simulink model "TBS_SIM"  (R2016b)
settings: Solver=ode5  StartTime=15  StopTime=30  FixedStep=0.002  RelTol=1e-3
PreLoadFcn:
  | TBS_Cai_simu_init_20170316
InitFcn:
  | TBS_Cai_simu_init_20170214
StopFcn:
  | TBS_SIMULATION_LOG
undefined symbols (not defined in the file): air_density, L1X, L2X, L3X, L3Y, MAC1, MAC2, MAC3, magnitude, motor_m0, motor_t0, ORIGIN_CD, ORIGIN_CL, ORIGIN_CM, S_seg1, S_seg2, S_seg3, y_ac
libraries: aerolibconvert2 x20, simulink x13, aerolibtransform2 x4, aerolibwind2 x3, aerolib6dof2 x1, aerolibasang x1
(part 1 of 2)
Description:
  | Combined hover/cruise/transition controller to Variant Control System
settings Model: Creator=SUN Jingxuan  LastModifiedBy=SUN Jingxuan
settings Model: ModifiedComment=|
  | SUN Jingxuan -- Fri Mar 10 21:29:21 2017 -- Version 2.0.29
  | revised distance from T to cg
settings Model: ModifiedHistory=|
  | SUN Jingxuan -- Fri Mar 10 21:29:21 2017 -- Version 2.0.29
  | revised distance from T to cg
  | 
  | SUN Jingxuan -- Fri Mar 10 21:07:47 2017 -- Version 2.0.28
  | add pid cruise controller
  | 
  | SUN Jingxuan -- Fri Mar 10 20:09:58 2017 -- Version 2.0.27
  | 
  | 
  | SUN Jingxuan -- Fri Mar 10 19:59:34 2017 -- Version 2.0.26
  | moment problem
  | 
  | SUN Jingxuan -- Thu Feb 16 15:35:11 2017 -- Version 2.0.25
  | Combined controller
  | 
  | SUN Jingxuan -- Thu Feb 16 14:30:29 2017 -- Version 2.0.24
  | add log of transition mode;
  | 
  | SUN Jingxuan -- Thu Feb 16 14:23:45 2017 -- Version 2.0.23
  | Resivised desired pitch angle of transition controller;
  | Delete y position and velocity control in transition;
  | Revise the Pitch angle criterionof changing to cruise controller
  | 
  | SUN Jingxuan -- Wed Feb 15 20:51:37 2017 -- Version 2.0.22
  | delete separate controller
  | 
  | SUN Jingxuan -- Wed Feb 15 20:47:11 2017 -- Version 2.0.21
  | Transition Controller
  | 
  | SUN Jingxuan -- Wed Feb 15 20:29:23 2017 -- Version 2.0.20
  | Transition pre test hover controller
  | 
  | SUN Jingxuan -- Wed Feb 15 15:19:36 2017 -- Version 2.0.19
  | Add Kp Yaw control
  | 
  | SUN Jingxuan -- Wed Feb 15 15:06:32 2017 -- Version 2.0.18
  | Revise Cruise controller
  | 
  | SUN Jingxuan -- Wed Feb 15 13:00:21 2017 -- Version 2.0.17
  | revised unit of AOA;
  | revised Cruise controller
  | 
  | SUN Jingxuan -- Wed Feb 15 11:23:14 2017 -- Version 2.0.7
  | Use Variant Controller Subsystem
  | Add Cruise Controller
  | 
  | SUN Jingxuan -- Wed Feb 15 11:23:14 2017 -- Version 2.0.7
  | Use Variant Controller Subsystem
  | Add Cruise Controller
  | 
  | SUN Jingxuan -- Wed Feb 15 11:23:14 2017 -- Version 2.0.7
  | Use Variant Controller Subsystem
  | Add Cruise Controller
  | 
  | SUN Jingxuan -- Wed Feb 15 11:23:14 2017 -- Version 2.0.7
  | Use Variant Controller Subsystem
  | Add Cruise Controller
  | 
  | SUN Jingxuan -- Wed Feb 15 11:23:14 2017 -- Version 2.0.7
  | Use Variant Controller Subsystem
  | Add Cruise Controller
  | 
  | SUN Jingxuan -- Wed Feb 15 11:23:14 2017 -- Version 2.0.7
  | Use Variant Controller Subsystem
  | Add Cruise Controller
  | 
  | SUN Jingxuan -- Wed Feb 15 11:23:14 2017 -- Version 2.0.7
  | Use Variant Controller Subsystem
  | Add Cruise Controller
  | 
  | SUN Jingxuan -- Wed Feb 15 11:23:14 2017 -- Version 2.0.7
  | Use Variant Controller Subsystem
  | Add Cruise Controller
  | 
  | SUN Jingxuan -- Wed Feb 15 11:23:14 2017 -- Version 2.0.7
  | Use Variant Controller Subsystem
  | Add Cruise Controller
  | 
  | SUN Jingxuan -- Wed Feb 15 11:23:14 2017 -- Version 2.0.7
  | Use Variant Controller Subsystem
  | Add Cruise Controller
  | 
  | SUN Jingxuan -- Tue Feb 14 21:13:32 2017 -- Version 2.0.5
  | Cruise controller test
  | 
  | SUN Jingxuan -- Tue Feb 14 21:13:32 2017 -- Version 2.0.5
  | Cruise controller test
  | 
  | SUN Jingxuan -- Tue Feb 14 19:41:26 2017 -- Version 2.0.4
  | Add result Log function
  | 
  | 
  | SUN Jingxuan -- Tue Feb 14 19:07:29 2017 -- Version 2.0.3
  | correct the side of the deflection of hovering controller
  | 
  | SUN Jingxuan -- Tue Feb 14 19:02:05 2017 -- Version 2.2
  | revised Actuators from elevator/Alieron to delta right/left

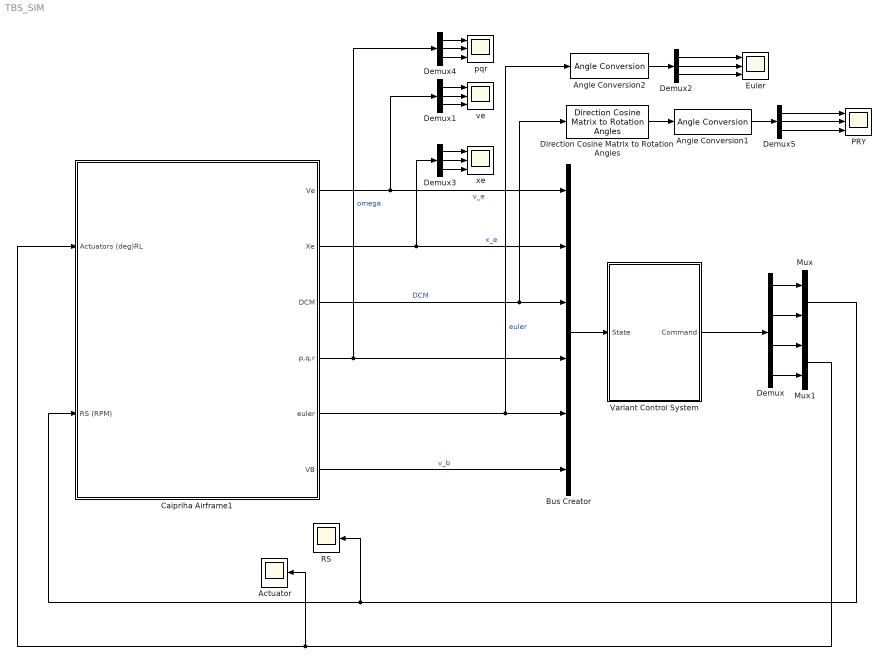
== system TBS_SIM ==
  Actuator : Scope
  Angle Conversion1 : aerolibconvert2/Angle Conversion  IU=rad  OU=deg
  Angle Conversion2 : aerolibconvert2/Angle Conversion  IU=rad  OU=deg
  Bus Creator : BusCreator  Inputs=6
  Caipriha Airframe1 : Subsystem
  Demux : Demux
  Demux{1..5} (5 alike) : Demux  Outputs=3
  Direction Cosine Matrix to Rotation Angles : aerolibtransform2/Direction Cosine Matrix to Rotation Angles  rotationOrder=YZX  lim=Default
      settings: AttributesFormatString=Rotation Order: %<rotationOrder>
  Euler : Scope  NumInputPorts=3
  Mux : Mux  Inputs=2
  Mux1 : Mux  Inputs=2
  PRY : Scope  NumInputPorts=3
  RS : Scope
  Variant Control System : Subsystem  Variant=on  OverrideUsingVariant=HoverYaw  PropagateVariantConditions=on
  pqr : Scope  NumInputPorts=3
  ve : Scope  NumInputPorts=3
  xe : Scope  NumInputPorts=3
  wires:
  Mux/1 -> Caipriha Airframe1/2(RS (RPM)), RS/1
  Mux1/1 -> Caipriha Airframe1/1(Actuators (deg)RL), Actuator/1
  Caipriha Airframe1/6("VB ") -> Bus Creator/6  "v_b"
  Demux3/1 -> xe/1
  Demux3/3 -> xe/3
  Demux3/2 -> xe/2
  Caipriha Airframe1/2(Xe) -> Bus Creator/2, Demux3/1  "x_e"
  Demux1/3 -> ve/3
  Caipriha Airframe1/1(Ve) -> Bus Creator/1, Demux1/1  "v_e"
  Demux1/2 -> ve/2
  Demux1/1 -> ve/1
  Angle Conversion1/1 -> Demux5/1
  Demux5/2 -> PRY/2
  Demux5/3 -> PRY/3
  Demux5/1 -> PRY/1
  Caipriha Airframe1/3(DCM) -> Bus Creator/3, Direction Cosine Matrix to Rotation Angles/1  "DCM"
  Angle Conversion2/1 -> Demux2/1
  Demux2/2 -> Euler/2
  Demux2/3 -> Euler/3
  Demux2/1 -> Euler/1
  Caipriha Airframe1/5(euler) -> Bus Creator/5, Angle Conversion2/1  "euler"
  Direction Cosine Matrix to Rotation Angles/1 -> Angle Conversion1/1
  Demux4/3 -> pqr/3
  Caipriha Airframe1/4(p,q,r) -> Bus Creator/4, Demux4/1  "omega"
  Demux4/2 -> pqr/2
  Demux4/1 -> pqr/1
  Bus Creator/1 -> Variant Control System/1(State)
  Demux/3 -> Mux1/1
  Demux/4 -> Mux1/2
  Demux/2 -> Mux/2
  Demux/1 -> Mux/1
  Variant Control System/1(Command) -> Demux/1

== system TBS_SIM/Caipriha Airframe1 ==
  Actuators (deg)RL : Inport
  RS (RPM) : Inport  Port=2
  6DOF (Quaternion) : aerolib6dof2/6DOF (Euler Angles)  units=Metric (MKS)  mtype=Fixed  rep=Quaternion  xme_0=init_pos_hov  Vm_0=init_vel_hov  eul_0=init_att_hov  pm_0=[0 0 0]  mass_0=0.876  mass_e=0.5  mass_f=2.0  inertia=Inertia  inertia_e=eye(3)  inertia_f=2*eye(3)  k_quat=1.0  vre_flag=on
  Aerodynamic Coefficient : Subsystem
  Alpha,Beta,Mach : Subsystem  AncestorBlock=aeroblk_lib_HL20/HL20 Airframe/Alpha,Beta,Mach
  Angle Conversion : aerolibconvert2/Angle Conversion  IU=rad  OU=deg
  Constant2 : Constant  Value=8.541
  Display2 : Display
  Environment Models1 : Subsystem  AncestorBlock=aeroblk_lib_HL20/HL20 Airframe/Environment Models
  Force&Moments : Subsystem
  Scope : Scope
  Terminator1 : Terminator  Commented=on
  Terminator2 : Terminator  Commented=on
  "Thrust " : Subsystem
  Ve : Outport  InitialOutput=0
  Xe : Outport  Port=2  InitialOutput=0
  DCM : Outport  Port=3  InitialOutput=0
  p,q,r : Outport  Port=4  InitialOutput=0
  euler : Outport  Port=5  InitialOutput=0
  "VB " : Outport  Port=6  InitialOutput=0
  wires:
  6DOF (Quaternion)/5 -> "VB "/1, Alpha,Beta,Mach/2(Vb)
  6DOF (Quaternion)/1 -> Environment Models1/1(Ve), Ve/1
  Constant2/1 -> Force&Moments/5(Gravity)
  6DOF (Quaternion)/4 -> Environment Models1/3(DCM), DCM/1, Force&Moments/6(DCM)
  6DOF (Quaternion)/3 -> euler/1
  Alpha,Beta,Mach/3(V_aircraft) -> Aerodynamic Coefficient/4(V), "Thrust "/2("AS ")
  Alpha,Beta,Mach/2(Incid) -> Angle Conversion/1, Aerodynamic Coefficient/5(Incid)
  "Thrust "/2(MT1) -> Force&Moments/2(MT)
  "Thrust "/1(F_T) -> Force&Moments/1("FT ")
  "Thrust "/4(T2) -> Aerodynamic Coefficient/2(T2)
  "Thrust "/3(T1) -> Aerodynamic Coefficient/1("T1 ")
  Aerodynamic Coefficient/2(M) -> Force&Moments/4(M)
  Aerodynamic Coefficient/1(F) -> Force&Moments/3(F)
  RS (RPM)/1 -> "Thrust "/1(RS1)
  Actuators (deg)RL/1 -> Aerodynamic Coefficient/3(Actuators)
  Environment Models1/1(Wind Velocity) -> Alpha,Beta,Mach/1(Wind Velocity)
  6DOF (Quaternion)/7 -> Terminator2/1
  6DOF (Quaternion)/6 -> p,q,r/1
  6DOF (Quaternion)/2 -> Environment Models1/2(Position), Xe/1
  6DOF (Quaternion)/8 -> Terminator1/1
  Force&Moments/2(LMN) -> 6DOF (Quaternion)/2
  Force&Moments/1(X,Y,Z) -> 6DOF (Quaternion)/1
  Alpha,Beta,Mach/1("[Vb]_total") -> Aerodynamic Coefficient/6(Vb_total)
  Angle Conversion/1 -> Scope/1, Display2/1

== system TBS_SIM/Variant Control System ==
  note: 1) Add Subsystem or Model blocks as valid variant choices.
      | 2) You cannot connect blocks at this level. At simulation, connectivity is automatically
      | determined, based on the active variant and port name matching.
  State : Inport
  Cruise : Subsystem  VariantControl=Cruise
  Hover : Subsystem  VariantControl=Hover
  Hover_yaw : Subsystem  VariantControl=HoverYaw
  PIDcruise : Subsystem  VariantControl=PIDcruise
  Transition : Subsystem  VariantControl=Transition
  Command : Outport

== system TBS_SIM/Caipriha Airframe1/Aerodynamic Coefficient ==
  "T1 " : Inport
  T2 : Inport  Port=2
  Actuators : Inport  Port=3
  V : Inport  Port=4
  Incid : Inport  Port=5
  Vb_total : Inport  Port=6
  Add : Sum  Inputs=++++
  Add1 : Sum  Inputs=++++
  DocBlock : simulink/Model-Wide Utilities/DocBlock  DocumentType=Text
      content=|
      | Segment definition: F:\MATLAB\TBS dynamic\segment.png
  Scope{,1..7} (8 alike) : Scope
  Segment1 : Subsystem
  Segment2 : Subsystem
  Segment3L1 : Subsystem
  Segment3R : Subsystem
  Selector : Selector  InputPortWidth=3  IndexOptions=Index vector (dialog)  Indices=[3]  OutputSizes=1
  Selector1 : Selector  InputPortWidth=2  IndexOptions=Index vector (dialog)  Indices=[1]  OutputSizes=1
  F : Outport
  M : Outport  Port=2
  wires:
  T2/1 -> Segment2/3(T2)
  "T1 "/1 -> Segment2/2("T1 ")
  Selector1/1 -> Segment3L1/1(alfa), Segment3R/1(alfa), Segment1/1(alfa), Segment2/1(alfa)
  Incid/1 -> Selector1/1
  Actuators/1 -> Segment3L1/3("actuatorsRL(deg) "), Segment3R/3("actuatorsRL(deg) "), Segment2/5("actuatorsRL(deg) ")
  V/1 -> Segment3L1/2(Airspeed), Segment3R/2(Airspeed), Segment1/2(Airspeed), Segment2/4(V)
  Selector/1 -> Segment2/6(Vb_z)
  Vb_total/1 -> Selector/1
  Segment2/1(F(3*1)) -> Scope/1, Add/1
  Segment1/1(F(3*1)) -> Scope1/1, Add/2
  Segment3R/1(F(3*1)1) -> Add/3, Scope2/1
  Segment3L1/1(F(3*1)) -> Scope3/1, Add/4
  Add/1 -> F/1
  Add1/1 -> M/1
  Segment2/2(M(3*1)) -> Scope4/1, Add1/1
  Segment1/2(Mcg(3*1)) -> Add1/2, Scope5/1
  Segment3R/2(Mcg(3*1)) -> Scope6/1, Add1/3
  Segment3L1/2(Mcg(3*1)) -> Scope7/1, Add1/4

== system TBS_SIM/Caipriha Airframe1/Alpha,Beta,Mach ==
  Wind Velocity : Inport  PortDimensions=3
  Vb : Inport  Port=2  PortDimensions=3
  "Incidence, Sideslip & Airspeed" : aerolibasang/Incidence, Sideslip, & Airspeed
  Mux : Mux  Inputs=2
  Sum : Sum  Inputs=|+-  SaturateOnIntegerOverflow=on  InputSameDT=on  OutDataTypeStr=Inherit: Same as first input
  "[Vb]_total" : Outport
  Incid : Outport  Port=2
  V_aircraft : Outport  Port=3
  wires:
  Sum/1 -> "[Vb]_total"/1, "Incidence, Sideslip & Airspeed"/1
  Wind Velocity/1 -> Sum/2
  "Incidence, Sideslip & Airspeed"/1 -> Mux/1  "Alpha"
  Mux/1 -> Incid/1
  "Incidence, Sideslip & Airspeed"/2 -> Mux/2  "Beta"
  Vb/1 -> Sum/1
  "Incidence, Sideslip & Airspeed"/3 -> V_aircraft/1

== system TBS_SIM/Caipriha Airframe1/Environment Models1 ==
  Ve : Inport
  Position : Inport  Port=2
  DCM : Inport  Port=3
  Abs : Abs
  Discrete Wind Gust Model : aerolibwind2/Discrete Wind Gust Model  units=Metric (MKS)  Gx=on  Gy=on  Gz=on  t_0=30  d_m=[100 100 100]  v_m=[1 1 1]
  Dot Product : DotProduct  SaturateOnIntegerOverflow=on  OutDataTypeStr=Inherit: Inherit via internal rule
  Horizontal Wind Model1 : aerolibwind2/Horizontal Wind Model  units=Metric (MKS)  Vw_source=Internal  Vwind=1  W_source=Internal  Wdeg=83
  Scope2 : Scope
  Selector : Selector  InputPortWidth=3  IndexOptions=Index vector (dialog)  Indices=[3]  OutputSizes=1
  Sum : Sum  Inputs=+++
  V : Math  Operator=sqrt  SaturateOnIntegerOverflow=on
  Wind Shear Model : aerolibwind2/Wind Shear Model  units=Metric (MKS)  phase=Other  W_20=0  Wdeg=0
  Wind Velocity : Outport  InitialOutput=0
  wires:
  V/1 -> Discrete Wind Gust Model/1
  Dot Product/1 -> V/1
  Ve/1 -> Dot Product/2, Dot Product/1
  Position/1 -> Selector/1
  Selector/1 -> Abs/1
  Abs/1 -> Wind Shear Model/1
  DCM/1 -> Horizontal Wind Model1/1, Wind Shear Model/2
  Wind Shear Model/1 -> Sum/2
  Discrete Wind Gust Model/1 -> Sum/1
  Sum/1 -> Scope2/1, Wind Velocity/1
  Horizontal Wind Model1/1 -> Sum/3

== system TBS_SIM/Caipriha Airframe1/Force&Moments ==
  "FT " : Inport
  MT : Inport  Port=2
  F : Inport  Port=3
  M : Inport  Port=4
  Gravity : Inport  Port=5
  DCM : Inport  Port=6
  Constant1 : Constant  Value=0
  Mux : Mux  Inputs=3
  Product : Product  Multiplication=Matrix(*)
  Sum : Sum  SaturateOnIntegerOverflow=on  InputSameDT=on  OutDataTypeStr=Inherit: Same as first input
  Sum1 : Sum
  Sum2 : Sum  Inputs=|++  SaturateOnIntegerOverflow=on  InputSameDT=on  OutDataTypeStr=Inherit: Same as first input
  X,Y,Z : Outport  InitialOutput=0
  LMN : Outport  Port=2  InitialOutput=0
  wires:
  Mux/1 -> Product/2
  Constant1/1 -> Mux/1, Mux/2
  Gravity/1 -> Mux/3
  DCM/1 -> Product/1
  Product/1 -> Sum2/2
  Sum2/1 -> X,Y,Z/1
  Sum/1 -> Sum2/1
  MT/1 -> Sum1/2
  "FT "/1 -> Sum/2
  Sum1/1 -> LMN/1
  M/1 -> Sum1/1
  F/1 -> Sum/1

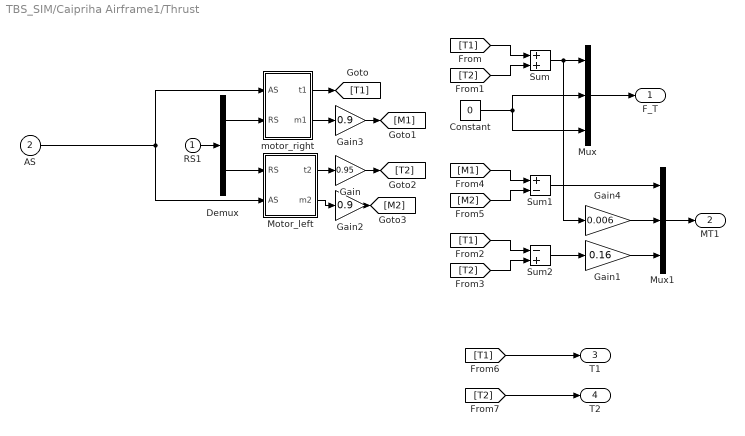
== system TBS_SIM/Caipriha Airframe1/Thrust  ==
  RS1 : Inport
  "AS " : Inport  Port=2
  Constant : Constant  Value=0
  Demux : Demux  Outputs=2
  Gain : Gain  Gain=0.95
  Gain1 : Gain  Gain=0.16
  Gain2 : Gain  Gain=0.9
  Gain3 : Gain  Gain=0.9
  Gain4 : Gain  Gain=0.006
  Motor_left : Subsystem
  Mux : Mux  Inputs=3
  Mux1 : Mux  Inputs=3
  Sum : Sum
  Sum1 : Sum  Inputs=+-
  Sum2 : Sum  Inputs=-+
  motor_right : Subsystem
  F_T : Outport
  MT1 : Outport  Port=2
  T1 : Outport  Port=3
  T2 : Outport  Port=4
  wires:
  Motor_left/2("m2 ") -> Gain2/1
  Gain3/1 -> [M1]
  Gain2/1 -> [M2]
  Gain/1 -> [T2]
  Motor_left/1(t2) -> Gain/1
  "AS "/1 -> Motor_left/2(AS), motor_right/1(AS)
  [T2] -> T2/1
  [T1] -> T1/1
  Gain4/1 -> Mux1/2
  [M2] -> Sum1/2
  [M1] -> Sum1/1
  [T2] -> Sum2/2
  [T1] -> Sum2/1
  [T2] -> Sum/2
  [T1] -> Sum/1
  motor_right/2("m1 ") -> Gain3/1
  motor_right/1(t1) -> [T1]
  Constant/1 -> Mux/2, Mux/3
  Sum1/1 -> Mux1/1
  Gain1/1 -> Mux1/3
  Sum2/1 -> Gain1/1
  Sum/1 -> Gain4/1, Mux/1
  Mux1/1 -> MT1/1
  Mux/1 -> F_T/1
  Demux/2 -> Motor_left/1(RS)
  Demux/1 -> motor_right/2(RS)
  RS1/1 -> Demux/1

== system TBS_SIM/Variant Control System/Cruise ==
  State : Inport
  Bus Selector : BusSelector  OutputSignals=v_e,x_e,DCM,omega,v_b,euler
  Cruise : Subsystem  VariantControl=CruseController
  Mux1 : Mux  Inputs=2
  "Command " : Outport
  wires:
  Mux1/1 -> "Command "/1
  Bus Selector/6 -> Cruise/6(Euler)  "<euler>"
  State/1 -> Bus Selector/1
  Cruise/1(RS) -> Mux1/1
  Cruise/2("Actuator ") -> Mux1/2
  Bus Selector/5 -> Cruise/5(V_b)  "<v_b>"
  Bus Selector/4 -> Cruise/4(pqr)  "<omega>"
  Bus Selector/3 -> Cruise/3(DCM)  "<DCM>"
  Bus Selector/2 -> Cruise/2(Xe)  "<x_e>"
  Bus Selector/1 -> Cruise/1(Ve)  "<v_e>"

== system TBS_SIM/Variant Control System/Hover ==
  State : Inport
  Attitude controller : Subsystem
  Bus Selector : BusSelector  OutputSignals=v_e,x_e,DCM,omega
  Constant : Constant  Value=[0,0,0]
  Constant1 : Constant  Value=[0,0,0]
  Demux4 : Demux
  Direction Cosine Matrix to Rotation Angles : aerolibtransform2/Direction Cosine Matrix to Rotation Angles  rotationOrder=YZX  lim=Default
      settings: AttributesFormatString=Rotation Order: %<rotationOrder>
  Mux2 : Mux
  Nav_controller(quad_axes) : Subsystem
  Saturation4 : Saturate  UpperLimit=10000  LowerLimit=0
  Saturation5 : Saturate  UpperLimit=10000  LowerLimit=0
  Saturation6 : Saturate  UpperLimit=20  LowerLimit=-20
  Saturation7 : Saturate  UpperLimit=20  LowerLimit=-20
  map1 : Subsystem
  Command : Outport
  wires:
  State/1 -> Bus Selector/1
  Saturation6/1 -> Mux2/3
  Constant/1 -> Nav_controller(quad_axes)/3(Desired velocity), Nav_controller(quad_axes)/4(Desired Position)
  map1/1(Act) -> Demux4/1
  Saturation4/1 -> Mux2/1
  Bus Selector/1 -> Nav_controller(quad_axes)/1(True velocity)  "<v_e>"
  Demux4/2 -> Saturation5/1
  Demux4/4 -> Saturation7/1
  Saturation7/1 -> Mux2/4
  Bus Selector/2 -> Nav_controller(quad_axes)/2(True Position)  "<x_e>"
  Demux4/1 -> Saturation4/1
  Saturation5/1 -> Mux2/2
  Bus Selector/3 -> Direction Cosine Matrix to Rotation Angles/1  "<DCM>"
  Nav_controller(quad_axes)/1(phi_des) -> Attitude controller/1(phi_des)
  Attitude controller/2("M_C ") -> map1/2(M_c)
  Demux4/3 -> Saturation6/1
  Bus Selector/4 -> Attitude controller/5(pqr)  "<omega>"
  Direction Cosine Matrix to Rotation Angles/1 -> Attitude controller/4(PRY), Nav_controller(quad_axes)/5(True PRY)
  Attitude controller/1(F_c) -> map1/1(F_c)
  Constant1/1 -> Attitude controller/6(des_pqr)
  Nav_controller(quad_axes)/3(F_des) -> Attitude controller/3(F_des)
  Nav_controller(quad_axes)/2("theta_des ") -> Attitude controller/2(theta_des)
  Mux2/1 -> Command/1

== system TBS_SIM/Variant Control System/Hover_yaw ==
  State : Inport
  Attitude controller : Subsystem
  Bus Selector : BusSelector  OutputSignals=v_e,x_e,DCM,omega
  Constant : Constant  Value=[0,0,0]
  Demux4 : Demux
  Direction Cosine Matrix to Rotation Angles : aerolibtransform2/Direction Cosine Matrix to Rotation Angles  rotationOrder=YZX  lim=Default
      settings: AttributesFormatString=Rotation Order: %<rotationOrder>
  Mux2 : Mux
  Nav_controller(quad_axes) : Subsystem
  Saturation4 : Saturate  UpperLimit=10000  LowerLimit=0
  Saturation5 : Saturate  UpperLimit=10000  LowerLimit=0
  Saturation6 : Saturate  UpperLimit=20  LowerLimit=-20
  Saturation7 : Saturate  UpperLimit=20  LowerLimit=-20
  Scope : Scope
  map1 : Subsystem
  Command : Outport
  wires:
  State/1 -> Bus Selector/1
  Saturation6/1 -> Mux2/3
  Constant/1 -> Nav_controller(quad_axes)/3(Desired velocity), Nav_controller(quad_axes)/4(Desired Position)
  map1/1(Act) -> Demux4/1
  Saturation4/1 -> Mux2/1
  Bus Selector/1 -> Nav_controller(quad_axes)/1(True velocity)  "<v_e>"
  Demux4/2 -> Saturation5/1
  Demux4/4 -> Saturation7/1
  Saturation7/1 -> Mux2/4
  Bus Selector/2 -> Nav_controller(quad_axes)/2(True Position)  "<x_e>"
  Demux4/1 -> Saturation4/1
  Saturation5/1 -> Mux2/2
  Bus Selector/3 -> Direction Cosine Matrix to Rotation Angles/1  "<DCM>"
  Nav_controller(quad_axes)/1(phi_des) -> Attitude controller/1(phi_des)
  Attitude controller/2("M_C ") -> Scope/1, map1/2(M_c)
  Demux4/3 -> Saturation6/1
  Direction Cosine Matrix to Rotation Angles/1 -> Attitude controller/4(PRY), Nav_controller(quad_axes)/5(True PRY)
  Attitude controller/1(F_c) -> map1/1(F_c)
  Nav_controller(quad_axes)/3(F_des) -> Attitude controller/3(F_des)
  Nav_controller(quad_axes)/2("theta_des ") -> Attitude controller/2(theta_des)
  Mux2/1 -> Command/1

== system TBS_SIM/Variant Control System/PIDcruise ==
  State : Inport
  Angle Conversion : aerolibconvert2/Angle Conversion  IU=rad  OU=deg
  Bus Selector : BusSelector  OutputSignals=euler,v_b
  Demux : Demux
  Mux1 : Mux  Inputs=2
  Mux2 : Mux  Inputs=2
  Mux3 : Mux  Inputs=2
  Saturation : Saturate  UpperLimit=10000  LowerLimit=0
  Saturation1 : Saturate  UpperLimit=10000  LowerLimit=0
  Saturation2 : Saturate  UpperLimit=16.5  LowerLimit=-23
  Saturation3 : Saturate  UpperLimit=16.5  LowerLimit=-23
  Subsystem : Subsystem
  Subsystem1 : Subsystem
  Subsystem2 : Subsystem
  "Command " : Outport
  wires:
  State/1 -> Bus Selector/1
  Bus Selector/1 -> Angle Conversion/1  "<euler>"
  Bus Selector/2 -> Subsystem1/1(Velocity)  "<v_b>"
  Subsystem2/1(Out1) -> Demux/1
  Saturation/1 -> Mux1/1
  Demux/1 -> Saturation/1
  Demux/2 -> Saturation1/1
  Saturation1/1 -> Mux1/2
  Saturation2/1 -> Mux3/1
  Demux/4 -> Saturation3/1
  Saturation3/1 -> Mux3/2
  Demux/3 -> Saturation2/1
  Mux1/1 -> Mux2/1
  Mux3/1 -> Mux2/2
  Mux2/1 -> "Command "/1
  Subsystem/1(Out1) -> Subsystem2/1(Moment)
  Subsystem1/1(Out1) -> Subsystem2/2(Fprce)
  Angle Conversion/1 -> Subsystem/1(Euler)

== system TBS_SIM/Variant Control System/Transition ==
  State : Inport
  Trans : Subsystem
  Command : Outport
  wires:
  State/1 -> Trans/1(State)
  Trans/1(Commands) -> Command/1

== system TBS_SIM/Caipriha Airframe1/Aerodynamic Coefficient/Segment1 ==
  alfa : Inport
  Airspeed : Inport  Port=2
  Add5 : Sum  Inputs=++|
  Constant1 : Constant  Value=0
  Constant2 : Constant  Value=0
  Constant3 : Constant  Value=0
  Gain11 : Gain  Gain=L1X
  Gain3 : Gain  Gain=-1
  Gain4 : Gain  Gain=-1
  Mux : Mux  Inputs=3
  Mux1 : Mux  Inputs=3
  right wing : Subsystem
  F(3*1) : Outport
  Mcg(3*1) : Outport  Port=2
  wires:
  Airspeed/1 -> right wing/1(v)
  Mux1/1 -> Mcg(3*1)/1
  Constant3/1 -> Mux1/3
  Add5/1 -> Mux1/2
  Mux/1 -> F(3*1)/1
  Constant1/1 -> Mux/2
  Gain3/1 -> Mux/3
  Gain4/1 -> Mux/1
  right wing/2(Fx) -> Gain4/1
  right wing/1(Fz) -> Gain3/1, Gain11/1
  Gain11/1 -> Add5/1
  right wing/3(Mac) -> Add5/2
  Constant2/1 -> Mux1/1
  alfa/1 -> right wing/2("ALFA ")

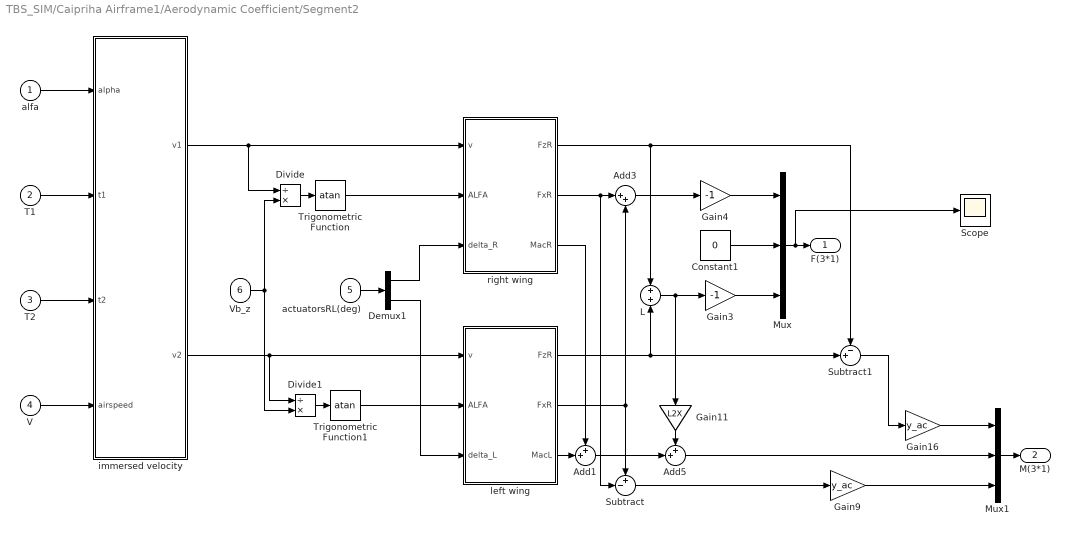
== system TBS_SIM/Caipriha Airframe1/Aerodynamic Coefficient/Segment2 ==
  alfa : Inport
  "T1 " : Inport  Port=2
  T2 : Inport  Port=3
  V : Inport  Port=4
  "actuatorsRL(deg) " : Inport  Port=5
  Vb_z : Inport  Port=6
  Add1 : Sum  Inputs=++|
  Add3 : Sum  Inputs=|++
  Add5 : Sum  Inputs=++|
  Constant1 : Constant  Value=0
  Demux1 : Demux  Outputs=2
  Divide : Product  Inputs=/*
  Divide1 : Product  Inputs=/*
  Gain11 : Gain  Gain=L2X
  Gain16 : Gain  Gain=y_ac
  Gain3 : Gain  Gain=-1
  Gain4 : Gain  Gain=-1
  Gain9 : Gain  Gain=y_ac
  L : Sum
  Mux : Mux  Inputs=3
  Mux1 : Mux  Inputs=3
  Scope : Scope
  Subtract : Sum  Inputs=+-|
  Subtract1 : Sum  Inputs=-+|
  Trigonometric Function : Trigonometry  Operator=atan  OutputSignalType=real
  Trigonometric Function1 : Trigonometry  Operator=atan
  immersed velocity : Subsystem
  left wing : Subsystem
  right wing : Subsystem
  F(3*1) : Outport
  M(3*1) : Outport  Port=2
  wires:
  V/1 -> immersed velocity/4(airspeed)
  immersed velocity/2(v2) -> left wing/1(v), Divide1/1
  immersed velocity/1(v1) -> right wing/1(v), Divide/1
  Mux1/1 -> M(3*1)/1
  Gain9/1 -> Mux1/3
  Add5/1 -> Mux1/2
  Subtract/1 -> Gain9/1
  Mux/1 -> Scope/1, F(3*1)/1
  Constant1/1 -> Mux/2
  Gain3/1 -> Mux/3
  Gain4/1 -> Mux/1
  Add3/1 -> Gain4/1
  L/1 -> Gain3/1, Gain11/1
  "actuatorsRL(deg) "/1 -> Demux1/1
  right wing/2(FxR) -> Subtract/2, Add3/1
  right wing/1(FzR) -> Subtract1/1, L/1
  T2/1 -> immersed velocity/3(t2)
  "T1 "/1 -> immersed velocity/2("t1 ")
  Vb_z/1 -> Divide1/2, Divide/2
  Divide/1 -> Trigonometric Function/1
  Divide1/1 -> Trigonometric Function1/1
  alfa/1 -> immersed velocity/1(alpha)
  left wing/2(FxR) -> Add3/2, Subtract/1
  left wing/3(MacL) -> Add1/2
  right wing/3(MacR) -> Add1/1
  left wing/1(FzR) -> Subtract1/2, L/2
  Gain11/1 -> Add5/1
  Add1/1 -> Add5/2
  Subtract1/1 -> Gain16/1
  Gain16/1 -> Mux1/1
  Demux1/1 -> right wing/3(delta_R)
  Demux1/2 -> left wing/3(delta_L)
  Trigonometric Function/1 -> right wing/2("ALFA ")
  Trigonometric Function1/1 -> left wing/2("ALFA ")

== system TBS_SIM/Caipriha Airframe1/Aerodynamic Coefficient/Segment3L1 ==
  alfa : Inport
  Airspeed : Inport  Port=2
  "actuatorsRL(deg) " : Inport  Port=3
  Constant1 : Constant  Value=0
  Gain1 : Gain  Gain=L3X
  Gain2 : Gain  Gain=-L3Y
  Gain3 : Gain  Gain=-1
  Gain4 : Gain  Gain=-1
  Gain5 : Gain  Gain=L3Y
  Mux : Mux  Inputs=3
  Mux1 : Mux  Inputs=3
  Selector : Selector  InputPortWidth=2  IndexOptions=Index vector (dialog)  Indices=[2]  OutputSizes=1
  Sum : Sum  Inputs=++|
  wing : Subsystem
  F(3*1) : Outport
  Mcg(3*1) : Outport  Port=2
  wires:
  Airspeed/1 -> wing/1(v)
  Mux1/1 -> Mcg(3*1)/1
  Gain2/1 -> Mux1/3
  wing/3(Mac) -> Sum/2
  Mux/1 -> F(3*1)/1
  Constant1/1 -> Mux/2
  Gain3/1 -> Mux/3
  Gain4/1 -> Mux/1
  wing/2(Fx) -> Gain2/1, Gain4/1
  wing/1(Fz) -> Gain1/1, Gain3/1, Gain5/1
  "actuatorsRL(deg) "/1 -> Selector/1
  Gain5/1 -> Mux1/1
  Selector/1 -> wing/3(delta_R)
  alfa/1 -> wing/2("ALFA ")
  Sum/1 -> Mux1/2
  Gain1/1 -> Sum/1

== system TBS_SIM/Caipriha Airframe1/Aerodynamic Coefficient/Segment3R ==
  alfa : Inport
  Airspeed : Inport  Port=2
  "actuatorsRL(deg) " : Inport  Port=3
  Constant4 : Constant  Value=0
  Gain1 : Gain  Gain=L3X
  Gain2 : Gain  Gain=L3Y
  Gain5 : Gain  Gain=-1
  Gain6 : Gain  Gain=-1
  Gain7 : Gain  Gain=-L3Y
  Mux2 : Mux  Inputs=3
  Mux3 : Mux  Inputs=3
  Selector : Selector  InputPortWidth=2  IndexOptions=Index vector (dialog)  Indices=[1]  OutputSizes=1
  Sum : Sum  Inputs=++|
  right wing : Subsystem
  F(3*1)1 : Outport
  Mcg(3*1) : Outport  Port=2
  wires:
  Airspeed/1 -> right wing/1(v)
  "actuatorsRL(deg) "/1 -> Selector/1
  Selector/1 -> right wing/3(delta_R)
  alfa/1 -> right wing/2("ALFA ")
  Mux3/1 -> Mcg(3*1)/1
  Gain2/1 -> Mux3/3
  right wing/3(MacR) -> Sum/2
  Mux2/1 -> F(3*1)1/1
  Constant4/1 -> Mux2/2
  Gain5/1 -> Mux2/3
  Gain6/1 -> Mux2/1
  right wing/2(FxR) -> Gain2/1, Gain6/1
  right wing/1(FzR) -> Gain1/1, Gain5/1, Gain7/1
  Gain7/1 -> Mux3/1
  Sum/1 -> Mux3/2
  Gain1/1 -> Sum/1

== system TBS_SIM/Caipriha Airframe1/Thrust /Motor_left ==
  RS : Inport
  AS : Inport  Port=2
  As_Prelookup : PreLookup  BreakpointsData=AS_R  ExtrapMethod=Linear
  M1LOOKUP1 : Interpolation_n-D  Table=motor_m0'  InternalRulePriority=Speed
  RS_Prelookup1 : PreLookup  BreakpointsData=RS  ExtrapMethod=Linear
  T1LOOKUP : Interpolation_n-D  Table=motor_t0'  InternalRulePriority=Speed
  t2 : Outport
  "m2 " : Outport  Port=2
  wires:
  RS/1 -> RS_Prelookup1/1
  AS/1 -> As_Prelookup/1
  M1LOOKUP1/1 -> "m2 "/1
  T1LOOKUP/1 -> t2/1
  RS_Prelookup1/2 -> T1LOOKUP/4, M1LOOKUP1/4
  RS_Prelookup1/1 -> M1LOOKUP1/3, T1LOOKUP/3
  As_Prelookup/2 -> T1LOOKUP/2, M1LOOKUP1/2
  As_Prelookup/1 -> T1LOOKUP/1, M1LOOKUP1/1

== system TBS_SIM/Caipriha Airframe1/Thrust /motor_right ==
  AS : Inport
  RS : Inport  Port=2
  As_Prelookup : PreLookup  BreakpointsData=AS_R  ExtrapMethod=Linear
  M1LOOKUP1 : Interpolation_n-D  Table=motor_m0'  InternalRulePriority=Speed
  RS_Prelookup1 : PreLookup  BreakpointsData=RS  ExtrapMethod=Linear
  T1LOOKUP : Interpolation_n-D  Table=motor_t0'  InternalRulePriority=Speed
  t1 : Outport
  "m1 " : Outport  Port=2
  wires:
  M1LOOKUP1/1 -> "m1 "/1
  T1LOOKUP/1 -> t1/1
  RS_Prelookup1/2 -> T1LOOKUP/4, M1LOOKUP1/4
  RS_Prelookup1/1 -> T1LOOKUP/3, M1LOOKUP1/3
  As_Prelookup/2 -> T1LOOKUP/2, M1LOOKUP1/2
  As_Prelookup/1 -> T1LOOKUP/1, M1LOOKUP1/1
  RS/1 -> RS_Prelookup1/1
  AS/1 -> As_Prelookup/1

== system TBS_SIM/Variant Control System/Cruise/Cruise ==
  Ve : Inport
  Xe : Inport  Port=2
  DCM : Inport  Port=3
  pqr : Inport  Port=4
  V_b : Inport  Port=5
  Euler : Inport  Port=6
  Angle Conversion : aerolibconvert2/Angle Conversion  IU=rad  OU=deg
  Demux : Demux
  Demux2 : Demux  Outputs=3
  Mux1 : Mux  Inputs=2
  Mux3 : Mux  Inputs=2
  Saturation : Saturate  UpperLimit=10000  LowerLimit=0
  Saturation1 : Saturate  UpperLimit=10000  LowerLimit=0
  Saturation2 : Saturate  UpperLimit=16.5  LowerLimit=-23
  Saturation3 : Saturate  UpperLimit=16.5  LowerLimit=-23
  Terminator : Terminator
  map : MATLAB Function  TreatAsAtomicUnit=on
  nav : MATLAB Function  TreatAsAtomicUnit=on
  ve : Scope  NumInputPorts=3
  RS : Outport
  "Actuator " : Outport  Port=2
  wires:
  V_b/1 -> nav/3(v)
  map/1(output) -> Demux/1
  Saturation/1 -> Mux1/1
  Demux/1 -> Saturation/1
  Demux/2 -> Saturation1/1
  Saturation1/1 -> Mux1/2
  Saturation2/1 -> Mux3/1
  Demux/4 -> Saturation3/1
  Saturation3/1 -> Mux3/2
  Demux/3 -> Saturation2/1
  nav/1(output) -> map/1(F_des)
  Angle Conversion/1 -> nav/2(PRY)
  Demux2/1 -> ve/1
  Demux2/2 -> ve/2
  Demux2/3 -> ve/3
  Ve/1 -> Demux2/1
  Xe/1 -> nav/1(p)
  pqr/1 -> nav/4(pqr)
  Mux1/1 -> RS/1
  Mux3/1 -> "Actuator "/1
  Euler/1 -> Angle Conversion/1
  DCM/1 -> Terminator/1

== system TBS_SIM/Variant Control System/Hover/Attitude controller ==
  phi_des : Inport
  theta_des : Inport  Port=2
  F_des : Inport  Port=3
  PRY : Inport  Port=4
  pqr : Inport  Port=5
  des_pqr : Inport  Port=6
  Add : Sum  Inputs=+-+
  Angle Conversion1 : aerolibconvert2/Angle Conversion  IU=rad  OU=deg
  Constant : Constant  Commented=on  Value=0
  Constant1 : Constant  Value=90
  Demux : Demux  Outputs=3
  Gain : Gain  Gain=[-0.05;0.07;0.08]
  Gain1 : Gain  Gain=[-0.4;-0.8;1.4]
  Gain2 : Gain  Gain=[0 0 1; 0 1 0; 1 0 0]  Multiplication=Matrix(K*u)
  Gain3 : Gain  Gain=-1
  Gain4 : Gain  Gain=-1
  Mux : Mux  Inputs=3
  Mux1 : Mux  Commented=on  Inputs=3
  Scope1 : Scope
  Scope2 : Scope
  Uniform Random Number : UniformRandomNumber  Commented=on  Minimum=-0.05  Maximum=0.05  SampleTime=0.005
  error_phi : Sum  Inputs=-+
  error_phi1 : Sum  Inputs=-+
  error_pqr : Sum  Inputs=-+
  error_pqr1 : Sum  Inputs=-+
  F_c : Outport
  "M_C " : Outport  Port=2
  wires:
  F_des/1 -> F_c/1
  des_pqr/1 -> error_pqr/1
  pqr/1 -> error_pqr/2
  phi_des/1 -> error_phi/1
  theta_des/1 -> error_phi1/1
  error_phi1/1 -> Mux/2
  Gain/1 -> Add/1
  Gain1/1 -> Scope2/1, Add/2
  PRY/1 -> Angle Conversion1/1
  error_phi/1 -> Mux/1
  Gain4/1 -> Mux/3
  Mux/1 -> Scope1/1, Gain/1
  error_pqr/1 -> Gain2/1
  Gain2/1 -> Gain1/1
  Add/1 -> "M_C "/1
  Demux/2 -> Gain3/1
  Gain3/1 -> error_phi/2
  Demux/1 -> error_pqr1/2
  Constant1/1 -> error_pqr1/1
  error_pqr1/1 -> error_phi1/2
  Angle Conversion1/1 -> Demux/1
  Demux/3 -> Gain4/1
  Uniform Random Number/1 -> Mux1/3
  Constant/1 -> Mux1/2, Mux1/1
  Mux1/1 -> Add/3

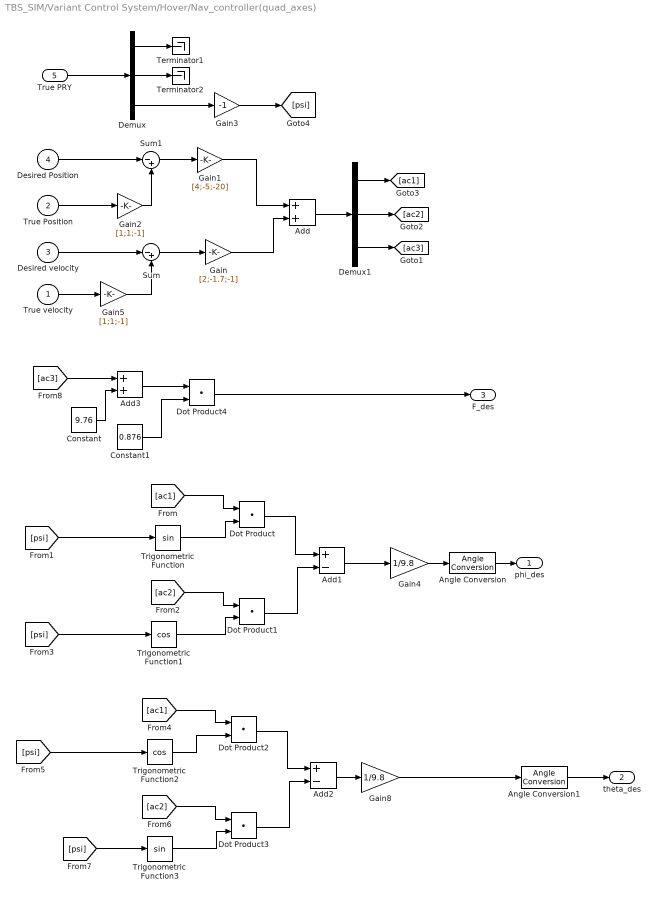
== system TBS_SIM/Variant Control System/Hover/Nav_controller(quad_axes) ==
  True velocity : Inport
  True Position : Inport  Port=2
  Desired velocity : Inport  Port=3
  Desired Position : Inport  Port=4
  True PRY : Inport  Port=5
  Add : Sum
  Add1 : Sum  Inputs=+-
  Add2 : Sum  Inputs=+-
  Add3 : Sum
  Angle Conversion : aerolibconvert2/Angle Conversion  IU=rad  OU=deg
  Angle Conversion1 : aerolibconvert2/Angle Conversion  IU=rad  OU=deg
  Constant : Constant  Value=9.76
  Constant1 : Constant  Value=0.876
  Demux : Demux  Outputs=3
  Demux1 : Demux  Outputs=3
  Dot Product{,1..4} (5 alike) : DotProduct  InputSameDT=on  OutDataTypeStr=Inherit: Inherit via internal rule
  Gain : Gain  Gain=[2;-1.7;-1]
  Gain1 : Gain  Gain=[4;-5;-20]
  Gain2 : Gain  Gain=[1;1;-1]
  Gain3 : Gain  Gain=-1
  Gain4 : Gain  Gain=1/9.8
  Gain5 : Gain  Gain=[1;1;-1]
  Gain8 : Gain  Gain=1/9.8
  Sum : Sum  Inputs=|-+
  Sum1 : Sum  Inputs=|-+
  Terminator1 : Terminator
  Terminator2 : Terminator
  Trigonometric Function : Trigonometry
  Trigonometric Function1 : Trigonometry  Operator=cos
  Trigonometric Function2 : Trigonometry  Operator=cos
  Trigonometric Function3 : Trigonometry
  phi_des : Outport
  "theta_des " : Outport  Port=2
  F_des : Outport  Port=3
  wires:
  True velocity/1 -> Gain5/1
  Desired velocity/1 -> Sum/1
  Sum/1 -> Gain/1
  Sum1/1 -> Gain1/1
  Gain1/1 -> Add/1
  Gain/1 -> Add/2
  True PRY/1 -> Demux/1
  Demux/1 -> Terminator1/1
  Demux/3 -> Gain3/1
  Demux/2 -> Terminator2/1
  Add/1 -> Demux1/1
  Demux1/2 -> [ac2]
  [ac1] -> Dot Product/1
  Trigonometric Function/1 -> Dot Product/2
  [psi] -> Trigonometric Function/1
  [ac2] -> Dot Product1/1
  Trigonometric Function1/1 -> Dot Product1/2
  [psi] -> Trigonometric Function1/1
  Dot Product/1 -> Add1/1
  Dot Product1/1 -> Add1/2
  Add1/1 -> Gain4/1
  [ac1] -> Dot Product2/1
  Trigonometric Function2/1 -> Dot Product2/2
  [psi] -> Trigonometric Function2/1
  [ac2] -> Dot Product3/1
  Trigonometric Function3/1 -> Dot Product3/2
  [psi] -> Trigonometric Function3/1
  Dot Product2/1 -> Add2/1
  Dot Product3/1 -> Add2/2
  Add2/1 -> Gain8/1
  [ac3] -> Add3/1
  Constant/1 -> Add3/2
  Add3/1 -> Dot Product4/1
  Constant1/1 -> Dot Product4/2
  Dot Product4/1 -> F_des/1
  Demux1/1 -> [ac1]
  Demux1/3 -> [ac3]
  True Position/1 -> Gain2/1
  Gain2/1 -> Sum1/2
  Desired Position/1 -> Sum1/1
  Gain3/1 -> [psi]
  Gain4/1 -> Angle Conversion/1
  Angle Conversion/1 -> phi_des/1
  Gain8/1 -> Angle Conversion1/1
  Angle Conversion1/1 -> "theta_des "/1
  Gain5/1 -> Sum/2

== system TBS_SIM/Variant Control System/Hover/map1 ==
  F_c : Inport
  M_c : Inport  Port=2
  Constant : Constant  Value=100
  Constant1 : Constant  Value=9.5
  Constant2 : Constant  Value=0.3
  Demux : Demux  Outputs=3
  Gain : Gain  Gain=1000
  Gain1 : Gain  Gain=1000
  Gain2 : Gain  Gain=50
  Gain3 : Gain  Gain=50
  Mux : Mux
  Sum : Sum  Inputs=-+|
  Sum1 : Sum  Inputs=|++
  Sum2 : Sum  Inputs=|+-
  Sum3 : Sum  Inputs=-+|
  Sum4 : Sum  Inputs=|++
  Sum5 : Sum  Inputs=|++
  Sum6 : Sum  Inputs=+-|
  Act : Outport
  wires:
  M_c/1 -> Demux/1
  F_c/1 -> Gain/1
  Demux/1 -> Gain1/1
  Gain1/1 -> Sum/2
  Constant/1 -> Sum/1
  Gain/1 -> Sum2/1, Sum1/1
  Sum/1 -> Sum1/2, Sum2/2
  Sum1/1 -> Mux/1
  Sum2/1 -> Mux/2
  Demux/2 -> Gain2/1
  Demux/3 -> Gain3/1
  Gain3/1 -> Sum4/1
  Constant1/1 -> Sum3/1
  Gain2/1 -> Sum3/2
  Constant2/1 -> Sum4/2
  Mux/1 -> Act/1
  Sum3/1 -> Sum5/1
  Sum4/1 -> Sum6/2, Sum5/2
  Sum5/1 -> Mux/4, Sum6/1
  Sum6/1 -> Mux/3

== system TBS_SIM/Variant Control System/Hover_yaw/Attitude controller ==
  phi_des : Inport
  theta_des : Inport  Port=2
  F_des : Inport  Port=3
  PRY : Inport  Port=4
  Angle Conversion1 : aerolibconvert2/Angle Conversion  IU=rad  OU=deg
  Constant1 : Constant  Value=90
  Demux : Demux  Outputs=3
  Gain3 : Gain  Gain=-1
  Mux1 : Mux  Inputs=3
  PID Controller : simulink/Continuous/PID Controller  Controller=PID  TimeDomain=Continuous-time  SampleTime=-1  IntegratorMethod=Forward Euler  FilterMethod=Forward Euler  Form=Parallel  UseFilter=on  ControllerParametersSource=internal  P=-15  I=-8  D=-8  N=20  InitialConditionSource=internal  InitialConditionForIntegrator=0  InitialConditionForFilter=0  ExternalReset=none  ZeroCross=off  LimitOutput=off  UpperSaturationLimit=inf  LowerSaturationLimit=-inf  LinearizeAsGain=on  AntiWindupMode=none  Kb=1  TrackingMode=off  Kt=1  PParamMin=[]  PParamMax=[]  IParamMin=[]  IParamMax=[]  DParamMin=[]  DParamMax=[]  NParamMin=[]  NParamMax=[]  KbParamMin=[]  KbParamMax=[]  KtParamMin=[]  KtParamMax=[]  POutMin=[]  POutMax=[]  IOutMin=[]  IOutMax=[]  DOutMin=[]  DOutMax=[]  NOutMin=[]  NOutMax=[]  KbOutMin=[]  KbOutMax=[]  KtOutMin=[]  KtOutMax=[]  IntegratorOutMin=[]  IntegratorOutMax=[]  FilterOutMin=[]  FilterOutMax=[]  SumOutMin=[]  SumOutMax=[]  SumI1OutMin=[]  SumI1OutMax=[]  SumI2OutMin=[]  SumI2OutMax=[]  SumI3OutMin=[]  SumI3OutMax=[]  SumDOutMin=[]  SumDOutMax=[]  SaturationOutMin=[]  SaturationOutMax=[]  IntegratorContinuousStateAttributes=''  IntegratorStateMustResolveToSignalObject=off  IntegratorRTWStateStorageClass=Auto  FilterContinuousStateAttributes=''  FilterStateMustResolveToSignalObject=off  FilterRTWStateStorageClass=Auto  DifferentiatorICPrevScaledInput=0  DifferentiatorOutMin=[]  DifferentiatorOutMax=[]
  PID Controller1 : simulink/Continuous/PID Controller  Controller=PID  TimeDomain=Continuous-time  SampleTime=-1  IntegratorMethod=Forward Euler  FilterMethod=Forward Euler  Form=Parallel  UseFilter=on  ControllerParametersSource=internal  P=-0.1  I=-0.05  D=-0.05  N=20  InitialConditionSource=internal  InitialConditionForIntegrator=0  InitialConditionForFilter=0  ExternalReset=none  ZeroCross=off  LimitOutput=off  UpperSaturationLimit=inf  LowerSaturationLimit=-inf  LinearizeAsGain=on  AntiWindupMode=none  Kb=1  TrackingMode=off  Kt=1  PParamMin=[]  PParamMax=[]  IParamMin=[]  IParamMax=[]  DParamMin=[]  DParamMax=[]  NParamMin=[]  NParamMax=[]  KbParamMin=[]  KbParamMax=[]  KtParamMin=[]  KtParamMax=[]  POutMin=[]  POutMax=[]  IOutMin=[]  IOutMax=[]  DOutMin=[]  DOutMax=[]  NOutMin=[]  NOutMax=[]  KbOutMin=[]  KbOutMax=[]  KtOutMin=[]  KtOutMax=[]  IntegratorOutMin=[]  IntegratorOutMax=[]  FilterOutMin=[]  FilterOutMax=[]  SumOutMin=[]  SumOutMax=[]  SumI1OutMin=[]  SumI1OutMax=[]  SumI2OutMin=[]  SumI2OutMax=[]  SumI3OutMin=[]  SumI3OutMax=[]  SumDOutMin=[]  SumDOutMax=[]  SaturationOutMin=[]  SaturationOutMax=[]  IntegratorContinuousStateAttributes=''  IntegratorStateMustResolveToSignalObject=off  IntegratorRTWStateStorageClass=Auto  FilterContinuousStateAttributes=''  FilterStateMustResolveToSignalObject=off  FilterRTWStateStorageClass=Auto  DifferentiatorICPrevScaledInput=0  DifferentiatorOutMin=[]  DifferentiatorOutMax=[]
  PID Controller2 : simulink/Continuous/PID Controller  Controller=PID  TimeDomain=Continuous-time  SampleTime=-1  IntegratorMethod=Forward Euler  FilterMethod=Forward Euler  Form=Parallel  UseFilter=on  ControllerParametersSource=internal  P=0.03  I=0.02  D=0.008  N=150  InitialConditionSource=internal  InitialConditionForIntegrator=0  InitialConditionForFilter=0  ExternalReset=none  ZeroCross=off  LimitOutput=off  UpperSaturationLimit=0.3  LowerSaturationLimit=0.3  LinearizeAsGain=on  AntiWindupMode=back-calculation  Kb=1  TrackingMode=off  Kt=1  PParamMin=[]  PParamMax=[]  IParamMin=[]  IParamMax=[]  DParamMin=[]  DParamMax=[]  NParamMin=[]  NParamMax=[]  KbParamMin=[]  KbParamMax=[]  KtParamMin=[]  KtParamMax=[]  POutMin=[]  POutMax=[]  IOutMin=[]  IOutMax=[]  DOutMin=[]  DOutMax=[]  NOutMin=[]  NOutMax=[]  KbOutMin=[]  KbOutMax=[]  KtOutMin=[]  KtOutMax=[]  IntegratorOutMin=[]  IntegratorOutMax=[]  FilterOutMin=[]  FilterOutMax=[]  SumOutMin=[]  SumOutMax=[]  SumI1OutMin=[]  SumI1OutMax=[]  SumI2OutMin=[]  SumI2OutMax=[]  SumI3OutMin=[]  SumI3OutMax=[]  SumDOutMin=[]  SumDOutMax=[]  SaturationOutMin=[]  SaturationOutMax=[]  IntegratorContinuousStateAttributes=''  IntegratorStateMustResolveToSignalObject=off  IntegratorRTWStateStorageClass=Auto  FilterContinuousStateAttributes=''  FilterStateMustResolveToSignalObject=off  FilterRTWStateStorageClass=Auto  DifferentiatorICPrevScaledInput=0  DifferentiatorOutMin=[]  DifferentiatorOutMax=[]
  Scope1 : Scope
  Scope3 : Scope
  Selector : Selector  InputPortWidth=3  IndexOptions=Index vector (dialog)  Indices=[3]  OutputSizes=1
  Terminator : Terminator
  error_phi : Sum  Inputs=-+
  error_phi1 : Sum  Inputs=-+
  error_pqr1 : Sum  Inputs=-+
  F_c : Outport
  "M_C " : Outport  Port=2
  wires:
  F_des/1 -> F_c/1
  phi_des/1 -> error_phi/1
  theta_des/1 -> error_phi1/1
  error_phi1/1 -> Scope1/1, PID Controller2/1
  Mux1/1 -> "M_C "/1
  Demux/2 -> Gain3/1
  Gain3/1 -> error_phi/2
  Demux/1 -> error_pqr1/2
  Constant1/1 -> error_pqr1/1
  error_pqr1/1 -> error_phi1/2
  Angle Conversion1/1 -> Demux/1
  Selector/1 -> PID Controller/1
  PID Controller/1 -> Mux1/3
  PID Controller2/1 -> Mux1/2
  PRY/1 -> Selector/1, Angle Conversion1/1
  error_phi/1 -> Scope3/1, PID Controller1/1
  PID Controller1/1 -> Mux1/1
  Demux/3 -> Terminator/1

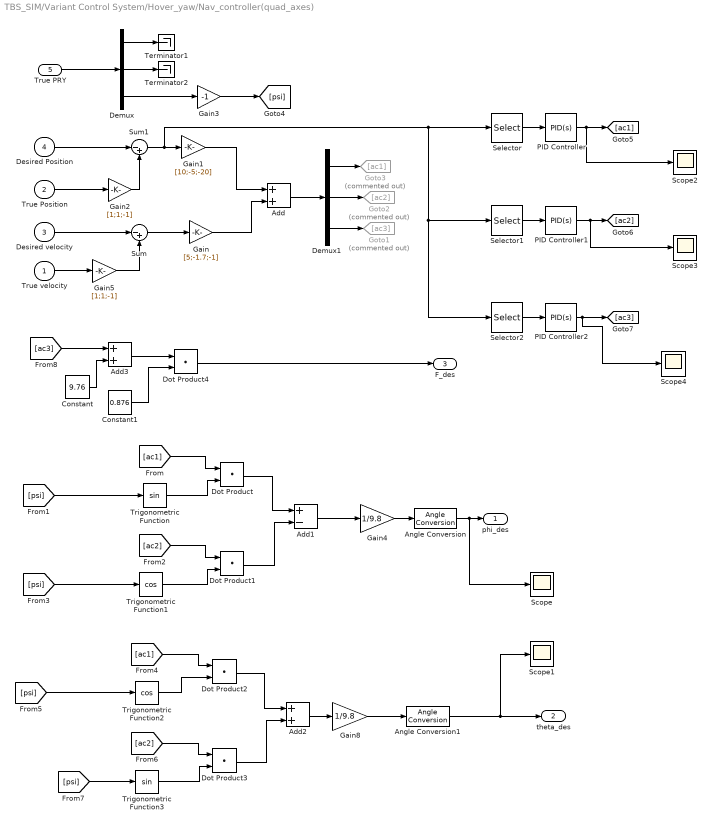
== system TBS_SIM/Variant Control System/Hover_yaw/Nav_controller(quad_axes) ==
  True velocity : Inport
  True Position : Inport  Port=2
  Desired velocity : Inport  Port=3
  Desired Position : Inport  Port=4
  True PRY : Inport  Port=5
  Add : Sum
  Add1 : Sum  Inputs=+-
  Add2 : Sum
  Add3 : Sum
  Angle Conversion : aerolibconvert2/Angle Conversion  IU=rad  OU=deg
  Angle Conversion1 : aerolibconvert2/Angle Conversion  IU=rad  OU=deg
  Constant : Constant  Value=9.76
  Constant1 : Constant  Value=0.876
  Demux : Demux  Outputs=3
  Demux1 : Demux  Outputs=3
  Dot Product{,1..4} (5 alike) : DotProduct  InputSameDT=on  OutDataTypeStr=Inherit: Inherit via internal rule
  Gain : Gain  Gain=[5;-1.7;-1]
  Gain1 : Gain  Gain=[10;-5;-20]
  Gain2 : Gain  Gain=[1;1;-1]
  Gain3 : Gain  Gain=-1
  Gain4 : Gain  Gain=1/9.8
  Gain5 : Gain  Gain=[1;1;-1]
  Gain8 : Gain  Gain=1/9.8
  Goto1 : Goto  Commented=on  GotoTag=ac3
  Goto2 : Goto  Commented=on  GotoTag=ac2
  Goto3 : Goto  Commented=on  GotoTag=ac1
  PID Controller : simulink/Continuous/PID Controller  Controller=PID  TimeDomain=Continuous-time  SampleTime=-1  IntegratorMethod=Forward Euler  FilterMethod=Forward Euler  Form=Parallel  UseFilter=on  ControllerParametersSource=internal  P=4  I=3  D=3  N=100  InitialConditionSource=internal  InitialConditionForIntegrator=0  InitialConditionForFilter=0  ExternalReset=none  LimitOutput=off  UpperSaturationLimit=inf  LowerSaturationLimit=-inf  LinearizeAsGain=on  AntiWindupMode=none  Kb=1  TrackingMode=off  Kt=1  PParamMin=[]  PParamMax=[]  IParamMin=[]  IParamMax=[]  DParamMin=[]  DParamMax=[]  NParamMin=[]  NParamMax=[]  KbParamMin=[]  KbParamMax=[]  KtParamMin=[]  KtParamMax=[]  POutMin=[]  POutMax=[]  IOutMin=[]  IOutMax=[]  DOutMin=[]  DOutMax=[]  NOutMin=[]  NOutMax=[]  KbOutMin=[]  KbOutMax=[]  KtOutMin=[]  KtOutMax=[]  IntegratorOutMin=[]  IntegratorOutMax=[]  FilterOutMin=[]  FilterOutMax=[]  SumOutMin=[]  SumOutMax=[]  SumI1OutMin=[]  SumI1OutMax=[]  SumI2OutMin=[]  SumI2OutMax=[]  SumI3OutMin=[]  SumI3OutMax=[]  SumDOutMin=[]  SumDOutMax=[]  SaturationOutMin=[]  SaturationOutMax=[]  IntegratorContinuousStateAttributes=''  IntegratorStateMustResolveToSignalObject=off  IntegratorRTWStateStorageClass=Auto  FilterContinuousStateAttributes=''  FilterStateMustResolveToSignalObject=off  FilterRTWStateStorageClass=Auto  DifferentiatorICPrevScaledInput=0  DifferentiatorOutMin=[]  DifferentiatorOutMax=[]
  PID Controller1 : simulink/Continuous/PID Controller  Controller=PID  TimeDomain=Continuous-time  SampleTime=-1  IntegratorMethod=Forward Euler  FilterMethod=Forward Euler  Form=Parallel  UseFilter=on  ControllerParametersSource=internal  P=-8  I=-4  D=-2  N=100  InitialConditionSource=internal  InitialConditionForIntegrator=0  InitialConditionForFilter=0  ExternalReset=none  LimitOutput=off  UpperSaturationLimit=inf  LowerSaturationLimit=-inf  LinearizeAsGain=on  AntiWindupMode=none  Kb=1  TrackingMode=off  Kt=1  PParamMin=[]  PParamMax=[]  IParamMin=[]  IParamMax=[]  DParamMin=[]  DParamMax=[]  NParamMin=[]  NParamMax=[]  KbParamMin=[]  KbParamMax=[]  KtParamMin=[]  KtParamMax=[]  POutMin=[]  POutMax=[]  IOutMin=[]  IOutMax=[]  DOutMin=[]  DOutMax=[]  NOutMin=[]  NOutMax=[]  KbOutMin=[]  KbOutMax=[]  KtOutMin=[]  KtOutMax=[]  IntegratorOutMin=[]  IntegratorOutMax=[]  FilterOutMin=[]  FilterOutMax=[]  SumOutMin=[]  SumOutMax=[]  SumI1OutMin=[]  SumI1OutMax=[]  SumI2OutMin=[]  SumI2OutMax=[]  SumI3OutMin=[]  SumI3OutMax=[]  SumDOutMin=[]  SumDOutMax=[]  SaturationOutMin=[]  SaturationOutMax=[]  IntegratorContinuousStateAttributes=''  IntegratorStateMustResolveToSignalObject=off  IntegratorRTWStateStorageClass=Auto  FilterContinuousStateAttributes=''  FilterStateMustResolveToSignalObject=off  FilterRTWStateStorageClass=Auto  DifferentiatorICPrevScaledInput=0  DifferentiatorOutMin=[]  DifferentiatorOutMax=[]
  PID Controller2 : simulink/Continuous/PID Controller  Controller=PID  TimeDomain=Continuous-time  SampleTime=-1  IntegratorMethod=Forward Euler  FilterMethod=Forward Euler  Form=Parallel  UseFilter=on  ControllerParametersSource=internal  P=-9  I=-5  D=-2  N=100  InitialConditionSource=internal  InitialConditionForIntegrator=0  InitialConditionForFilter=0  ExternalReset=none  LimitOutput=off  UpperSaturationLimit=inf  LowerSaturationLimit=-inf  LinearizeAsGain=on  AntiWindupMode=none  Kb=1  TrackingMode=off  Kt=1  PParamMin=[]  PParamMax=[]  IParamMin=[]  IParamMax=[]  DParamMin=[]  DParamMax=[]  NParamMin=[]  NParamMax=[]  KbParamMin=[]  KbParamMax=[]  KtParamMin=[]  KtParamMax=[]  POutMin=[]  POutMax=[]  IOutMin=[]  IOutMax=[]  DOutMin=[]  DOutMax=[]  NOutMin=[]  NOutMax=[]  KbOutMin=[]  KbOutMax=[]  KtOutMin=[]  KtOutMax=[]  IntegratorOutMin=[]  IntegratorOutMax=[]  FilterOutMin=[]  FilterOutMax=[]  SumOutMin=[]  SumOutMax=[]  SumI1OutMin=[]  SumI1OutMax=[]  SumI2OutMin=[]  SumI2OutMax=[]  SumI3OutMin=[]  SumI3OutMax=[]  SumDOutMin=[]  SumDOutMax=[]  SaturationOutMin=[]  SaturationOutMax=[]  IntegratorContinuousStateAttributes=''  IntegratorStateMustResolveToSignalObject=off  IntegratorRTWStateStorageClass=Auto  FilterContinuousStateAttributes=''  FilterStateMustResolveToSignalObject=off  FilterRTWStateStorageClass=Auto  DifferentiatorICPrevScaledInput=0  DifferentiatorOutMin=[]  DifferentiatorOutMax=[]
  Scope{,1..4} (5 alike) : Scope
  Selector : Selector  InputPortWidth=3  IndexOptions=Index vector (dialog)  Indices=[1]  OutputSizes=1
  Selector1 : Selector  InputPortWidth=3  IndexOptions=Index vector (dialog)  Indices=[2]  OutputSizes=1
  Selector2 : Selector  InputPortWidth=3  IndexOptions=Index vector (dialog)  Indices=[3]  OutputSizes=1
  Sum : Sum  Inputs=|-+
  Sum1 : Sum  Inputs=|-+
  Terminator1 : Terminator
  Terminator2 : Terminator
  Trigonometric Function : Trigonometry
  Trigonometric Function1 : Trigonometry  Operator=cos
  Trigonometric Function2 : Trigonometry  Operator=cos
  Trigonometric Function3 : Trigonometry
  phi_des : Outport
  "theta_des " : Outport  Port=2
  F_des : Outport  Port=3
  wires:
  True velocity/1 -> Gain5/1
  Desired velocity/1 -> Sum/1
  Sum/1 -> Gain/1
  Gain1/1 -> Add/1
  Gain/1 -> Add/2
  True PRY/1 -> Demux/1
  Demux/1 -> Terminator1/1
  Demux/3 -> Gain3/1
  Demux/2 -> Terminator2/1
  Add/1 -> Demux1/1
  Demux1/2 -> Goto2/1
  [ac1] -> Dot Product/1
  Trigonometric Function/1 -> Dot Product/2
  [psi] -> Trigonometric Function/1
  [ac2] -> Dot Product1/1
  Trigonometric Function1/1 -> Dot Product1/2
  [psi] -> Trigonometric Function1/1
  Dot Product/1 -> Add1/1
  Dot Product1/1 -> Add1/2
  Add1/1 -> Gain4/1
  [ac1] -> Dot Product2/1
  Trigonometric Function2/1 -> Dot Product2/2
  [psi] -> Trigonometric Function2/1
  [ac2] -> Dot Product3/1
  Trigonometric Function3/1 -> Dot Product3/2
  [psi] -> Trigonometric Function3/1
  Dot Product2/1 -> Add2/1
  Dot Product3/1 -> Add2/2
  Add2/1 -> Gain8/1
  [ac3] -> Add3/1
  Constant/1 -> Add3/2
  Add3/1 -> Dot Product4/1
  Constant1/1 -> Dot Product4/2
  Dot Product4/1 -> F_des/1
  Demux1/1 -> Goto3/1
  Demux1/3 -> Goto1/1
  True Position/1 -> Gain2/1
  Gain2/1 -> Sum1/2
  Desired Position/1 -> Sum1/1
  Gain3/1 -> [psi]
  Gain4/1 -> Angle Conversion/1
  Angle Conversion/1 -> Scope/1, phi_des/1
  Gain8/1 -> Angle Conversion1/1
  Angle Conversion1/1 -> Scope1/1, "theta_des "/1
  Gain5/1 -> Sum/2
  Selector/1 -> PID Controller/1
  PID Controller/1 -> Scope2/1, [ac1]
  Selector1/1 -> PID Controller1/1
  PID Controller1/1 -> Scope3/1, [ac2]
  Sum1/1 -> Selector2/1, Selector1/1, Selector/1, Gain1/1
  Selector2/1 -> PID Controller2/1
  PID Controller2/1 -> Scope4/1, [ac3]

== system TBS_SIM/Variant Control System/Hover_yaw/map1 ==
  F_c : Inport
  M_c : Inport  Port=2
  Constant : Constant  Value=100
  Constant1 : Constant  Value=9.5
  Constant2 : Constant  Value=0.3
  Demux : Demux  Outputs=3
  Gain : Gain  Gain=1000
  Gain1 : Gain  Gain=1000
  Gain2 : Gain  Gain=50
  Gain3 : Gain  Gain=50
  Mux : Mux
  Sum : Sum  Inputs=-+|
  Sum1 : Sum  Inputs=|++
  Sum2 : Sum  Inputs=|+-
  Sum3 : Sum  Inputs=-+|
  Sum4 : Sum  Inputs=|++
  Sum5 : Sum  Inputs=|++
  Sum6 : Sum  Inputs=+-|
  Act : Outport
  wires:
  M_c/1 -> Demux/1
  F_c/1 -> Gain/1
  Demux/1 -> Gain1/1
  Gain1/1 -> Sum/2
  Constant/1 -> Sum/1
  Gain/1 -> Sum2/1, Sum1/1
  Sum/1 -> Sum1/2, Sum2/2
  Sum1/1 -> Mux/1
  Sum2/1 -> Mux/2
  Demux/2 -> Gain2/1
  Demux/3 -> Gain3/1
  Gain3/1 -> Sum4/1
  Constant1/1 -> Sum3/1
  Gain2/1 -> Sum3/2
  Constant2/1 -> Sum4/2
  Mux/1 -> Act/1
  Sum3/1 -> Sum5/1
  Sum4/1 -> Sum6/2, Sum5/2
  Sum5/1 -> Mux/4, Sum6/1
  Sum6/1 -> Mux/3
